simulink model "vdc_r2022a"  (R2022a)
settings: Solver=VariableStepAuto  StartTime=0.0  StopTime=10.0  RelTol=1e-3
libraries: simulink x1
settings Model: Creator=no  LastModifiedBy=no
settings ModelReferenceCC: EnableRefExpFcnMdlSchedulingChecks=off
settings RTWCC: Description=Generic Real-Time Target

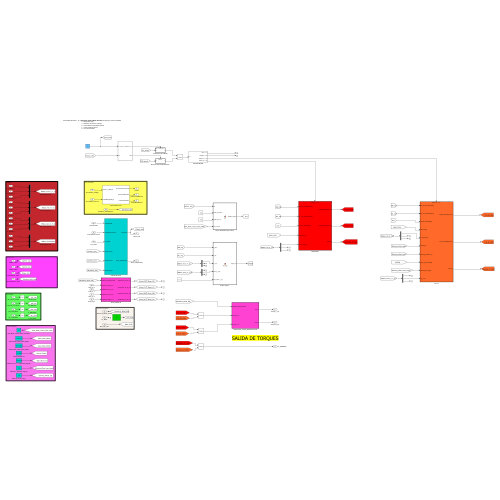
[thumbnail: Simulink's stored preview of the top-level diagram]
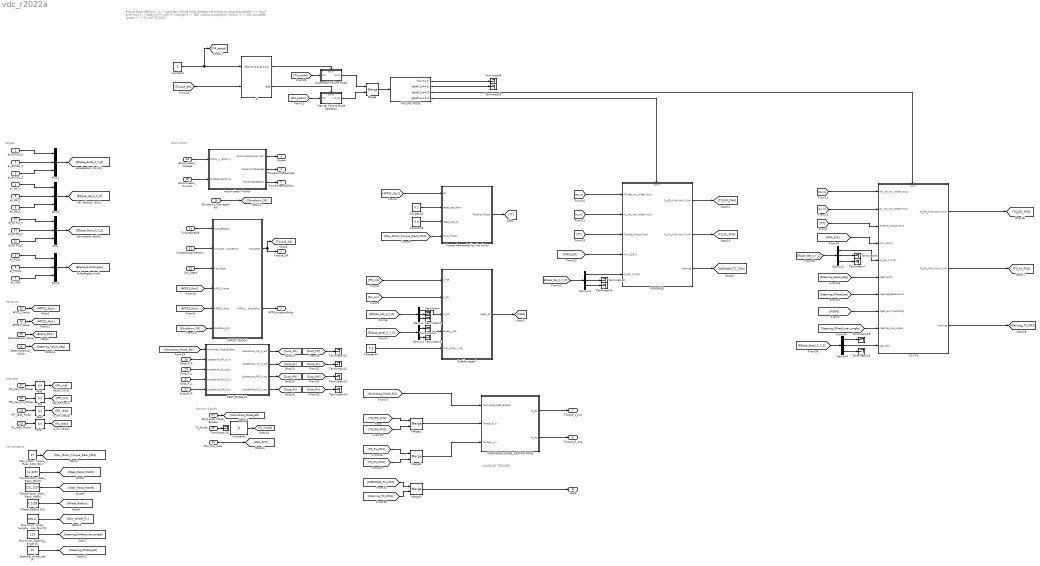
== system vdc_r2022a ==
  note: SALIDA DE TORQUES
  note: Ellipse
  note: Sensorics
  note: Velocities
  note: Car constants
  note: Failure Mode Selection: 5 -> Automatic Failure Mode Selection according to sensors available
      | 4 -> Rigid Axle (red)
      | 3 -> Steering TV with TC (orange)
      | 2 -> VDC without longitudinal (yellow)
      | 1 -> VDC complete (green)
      | 0 -> TV with TC 2023
  note: Accumulator
  note: Random Signals
  el_ACCEL_X : Inport
  el_ACCEL_Y : Inport  Port=2
  el_ACCEL_Z : Inport  Port=3
  el_Vel_X : Inport  Port=4
  el_Vel_Y : Inport  Port=5
  el_Vel_Z : Inport  Port=6
  el_YAW : Inport  Port=7
  el_PITCH : Inport  Port=8
  el_ROLL : Inport  Port=9
  el_GYRO_X : Inport  Port=10
  el_GYRO_Y : Inport  Port=11
  el_GYRO_Z : Inport  Port=12
  APPS2_Value : Inport  Port=13
  APPS1_Value : Inport  Port=14
  BrakeSensor_Value : Inport  Port=15
  SteeringSensor_Value : Inport  Port=16
  RL_Vel_ms_Wheel : Inport  Port=17
  RR_Vel_ms_Wheel : Inport  Port=18
  RR_rads_Motor : Inport  Port=19
  RL_rads_Motor : Inport  Port=20
  TorqueEnable : Inport  Port=21
  CriticalDisconnection : Inport  Port=22
  Car_State : Inport  Port=23
  Accumulator_Voltage : Inport  Port=24
  Accumulator_Current : Inport  Port=25
  Shutdown_PackageIntck : Inport  Port=26
  Workshop_Mode_Enable : Inport  Port=27
  TV_Mode : Inport  Port=28
  Susp_F_L : Inport  Port=29
  Susp_F_R : Inport  Port=30
  Susp_R_L : Inport  Port=31
  Susp_R_R : Inport  Port=32
  Max_slip_ratio : Inport  Port=33
  Abs{,1..3} (4 alike) : Abs  SaturateOnIntegerOverflow=off
  Accumulator Power : Subsystem
  Automatic Failure Mode : Subsystem  TreatAsAtomicUnit=on
  Constant : Constant  Value=5
  Constant1 : Constant  Value=3
  Constant2 : Constant  Value=0.2
  Constant3 : Constant  Value=0.8
  Constant4 : Constant  Value=7.5
  Demux{,1..4} (5 alike) : Demux  Outputs=3
  Enable regen? : MATLAB Function  TreatAsAtomicUnit=on
  FAILURE MODE : If  IfExpression=u1 == 1  ElseIfExpressions=u1 == 2, u1 == 3, u1 == 4  ShowElse=off
  If : If  NumInputs=2  IfExpression=u1 == 5 & u2 == 1
  Manual Failure Mode Selection : Subsystem  TreatAsAtomicUnit=on
  Max_Motor_Torque_Rear_FM4 [Nm] : Constant  Value=27
  Maximum_Force_Longitudinal_Slip [N] : Constant  Value=1364.44
  Maximum_Steering_angle [º] : Constant  Value=125
  Merge{,1..3} (4 alike) : Merge
  Mux{,1..3} (4 alike) : Mux  Inputs=3
  RIGIDAXLE : Subsystem
  SAFETY BLOCK : Subsystem
  Steering_wheel_sat [º] : Constant  Value=10
  TC+TV : Subsystem
  TEST_MODE_IN : Subsystem  TreatAsAtomicUnit=on
  Terminator{,1..16} (17 alike) : Terminator
  Torque demanded by the driver : MATLAB Function  TreatAsAtomicUnit=on
  Transmission_Gear_Ratio_MtoW : Constant  Value=11.3257
  Transmission_Gear_Ratio_WtoM : Constant  Value=1/11.3257
  WORKSHOP_MODE_RESTRICTIONS : Subsystem  TreatAsAtomicUnit=on
  Wheel_Radius [m] : Constant  Value=0.2285
  APPS_Implausibility : Outport  VectorParamsAs1DForOutWhenUnconnected=off
  Torque_OK : Outport  Port=2  VectorParamsAs1DForOutWhenUnconnected=off
  Power : Outport  Port=3  VectorParamsAs1DForOutWhenUnconnected=off
  PowerLimitReached : Outport  Port=4  VectorParamsAs1DForOutWhenUnconnected=off
  PowerMean500ms : Outport  Port=5  VectorParamsAs1DForOutWhenUnconnected=off
  Torque_R_out : Outport  Port=6
  Torque_L_out : Outport  Port=7
  Out3 : Outport  Port=8  SignalName=TC_WARNING
  wires:
  Torque demanded by the driver/1(Throttle_Torque) -> [TT]
  [TT] -> TC+TV/3(Throttle_Torque [Nm])
  Enable regen?/1(regen_en) -> [RGEN]
  [RGEN] -> TC+TV/8(regen_en [True/False])
  el_PITCH/1 -> Mux3/2
  el_GYRO_Z/1 -> Mux/3
  el_ACCEL_Y/1 -> Mux1/2
  Mux3/1 -> [Ellipse_EulerAngles]
  el_ROLL/1 -> Mux3/1
  Mux1/1 -> [Ellipse_Accel_X_Y_Z]
  el_YAW/1 -> Mux3/3
  el_Vel_X/1 -> Mux2/1
  Mux2/1 -> [Ellipse_Vel_X_Y_Z]
  el_GYRO_X/1 -> Mux/1
  el_Vel_Z/1 -> Mux2/3
  el_ACCEL_X/1 -> Mux1/1
  Mux/1 -> [Ellipse_Gyro_X_Y_Z]
  el_GYRO_Y/1 -> Mux/2
  el_ACCEL_Z/1 -> Mux1/3
  el_Vel_Y/1 -> Mux2/2
  SteeringSensor_Value/1 -> [Steering_Value_deg]
  APPS1_Value/1 -> [APPS1_0to1]
  BrakeSensor_Value/1 -> [Brake_0to1]
  APPS2_Value/1 -> [APPS2_0to1]
  [APPS1_0to1] -> Torque demanded by the driver/1(AP)
  Abs/1 -> [RR_ms]
  Abs2/1 -> [RR_rads]
  RR_Vel_ms_Wheel/1 -> Abs/1
  Abs1/1 -> [RL_ms]
  RR_rads_Motor/1 -> Abs2/1
  RL_rads_Motor/1 -> Abs3/1
  Abs3/1 -> [RL_rads]
  RL_Vel_ms_Wheel/1 -> Abs1/1
  Transmission_Gear_Ratio_MtoW/1 -> [Gear_Ratio_MtoW]
  Maximum_Force_Longitudinal_Slip [N]/1 -> [Max_Wheel_Fx]
  Transmission_Gear_Ratio_WtoM/1 -> [Gear_Ratio_WtoM]
  Wheel_Radius [m]/1 -> [Wheel_Radius]
  Max_Motor_Torque_Rear_FM4 [Nm]/1 -> [Max_Motor_Torque_Rear_FM4]
  [RR_ms] -> Enable regen?/1(V_RR)
  [RL_ms] -> Enable regen?/2(V_RL)
  [Ellipse_Vel_X_Y_Z] -> Demux/1
  Demux/1 -> Enable regen?/3(V_CG)
  Demux/2 -> Terminator/1
  Demux/3 -> Terminator1/1
  Demux1/3 -> Terminator3/1
  [Ellipse_Accel_X_Y_Z] -> Demux1/1
  Demux1/1 -> Terminator2/1
  Demux1/2 -> Enable regen?/4(accel_y_CG)
  [Max_Motor_Torque_Rear_FM4] -> Torque demanded by the driver/4(max_torque)
  Manual Failure Mode Selection/1(Out1) -> Merge/2
  If/2 -> Manual Failure Mode Selection/Action
  [FM_select] -> Manual Failure Mode Selection/1(In1)
  [TV_mode] -> Automatic Failure Mode/1(In1)
  Automatic Failure Mode/1(Out1) -> Merge/1
  Merge/1 -> FAILURE MODE/1
  Constant/1 -> [FM_select], If/1
  [APPS1_0to1] -> SAFETY BLOCK/4(APPS1_Value)
  SAFETY BLOCK/1(TorqueOK) -> Torque_OK/1, [Torque_OK]
  TorqueEnable/1 -> SAFETY BLOCK/1(TorqueEnable)
  SAFETY BLOCK/2(APPS_Implausibility) -> APPS_Implausibility/1
  [Shutdown_OK] -> SAFETY BLOCK/6(Shutdown_OK)
  [APPS2_0to1] -> SAFETY BLOCK/5(APPS2_Value)
  CriticalDisconnection/1 -> SAFETY BLOCK/2(CriticalDisconnection)
  Car_State/1 -> SAFETY BLOCK/3(Car_State)
  Accumulator Power/2(PowerLimitReached) -> PowerLimitReached/1
  Accumulator Power/1(AccumulatorPower [kW]) -> Power/1
  Accumulator Power/3(PowerMean500ms) -> PowerMean500ms/1
  Shutdown_PackageIntck/1 -> [Shutdown_OK]
  Accumulator_Voltage/1 -> Accumulator Power/1(TOTAL_V_BMS [V])
  Accumulator_Current/1 -> Accumulator Power/2(CURRENT_BMS [A])
  If/1 -> Automatic Failure Mode/Action
  FAILURE MODE/4 -> RIGIDAXLE/Action
  FAILURE MODE/3 -> TC+TV/Action
  FAILURE MODE/2 -> Terminator5/1
  FAILURE MODE/1 -> Terminator4/1
  Maximum_Steering_angle [º]/1 -> [Steering_Wheel_max_angle]
  Steering_wheel_sat [º]/1 -> [Steering_Wheel_sat]
  [Torque_OK] -> If/2
  [RR_ms] -> TC+TV/1(RR_Vel_ms_Wheel [m/s])
  [RL_ms] -> TC+TV/2(RL_Vel_ms_Wheel [m/s])
  [MAX_SLR] -> TC+TV/4(MAX_SLR [])
  [Steering_Value_deg] -> TC+TV/6(steering (º))
  [Steering_Wheel_sat] -> TC+TV/7(steering_deadzone (º))
  [Ellipse_Vel_X_Y_Z] -> Demux2/1
  Demux2/1 -> TC+TV/5(el_Vel_X [m/s])
  Demux2/2 -> Terminator6/1
  Demux2/3 -> Terminator7/1
  Demux3/3 -> Terminator9/1
  Demux3/2 -> Terminator8/1
  [Ellipse_Vel_X_Y_Z] -> Demux3/1
  Demux3/1 -> RIGIDAXLE/5(el_Vel_X [m/s])
  [RR_ms] -> RIGIDAXLE/1(RR_Vel_ms_Wheel [m/s])
  [TT] -> RIGIDAXLE/3(Throttle_Torque [Nm])
  [RL_ms] -> RIGIDAXLE/2(RL_Vel_ms_Wheel [m/s])
  [MAX_SLR] -> RIGIDAXLE/4(MAX_SLR [])
  RIGIDAXLE/1(Tq_RR_FM4 [Nm] (0,inf)) -> [TQ_RR_FM4]
  RIGIDAXLE/2(Tq_RL_FM4 [Nm] (0,inf)) -> [TQ_RL_FM4]
  TC+TV/1(Tq_RR_FM3 [Nm] (0,inf)) -> [TQ_RR_FM3]
  TC+TV/2(Tq_RL_FM3 [Nm] (0,inf)) -> [TQ_RL_FM3]
  [TQ_RR_FM4] -> Merge1/1
  [TQ_RR_FM3] -> Merge1/2
  [TQ_RL_FM4] -> Merge2/1
  [TQ_RL_FM3] -> Merge2/2
  Constant1/1 -> [TV_mode]
  Workshop_Mode_Enable/1 -> [Workshop_Mode_EN]
  TV_Mode/1 -> Terminator10/1
  TEST_MODE_IN/2(Suspension_FL_N_out) -> [Susp_FL]
  [Workshop_Mode_EN] -> TEST_MODE_IN/1(Workshop_Mode_Enable)
  Susp_F_R/1 -> TEST_MODE_IN/2(Suspension_FR_N_in)
  Susp_R_L/1 -> TEST_MODE_IN/4(Suspension_RL_N_in)
  Susp_R_R/1 -> TEST_MODE_IN/5(Suspension_RR_N_in)
  TEST_MODE_IN/3(Suspension_RR_N_out) -> [Susp_RR]
  Susp_F_L/1 -> TEST_MODE_IN/3(Suspension_FL_N_in)
  TEST_MODE_IN/4(Suspension_RL_N_out) -> [Susp_RL]
  TEST_MODE_IN/1(Suspension_FR_N_out) -> [Susp_FR]
  [Susp_FR] -> Terminator11/1
  [Susp_RL] -> Terminator14/1
  [Susp_RR] -> Terminator13/1
  [Susp_FL] -> Terminator12/1
  Constant2/1 -> Torque demanded by the driver/2(pedal_sat_down)
  Constant3/1 -> Torque demanded by the driver/3(pedal_sat_up)
  Constant4/1 -> Enable regen?/5(max_accel_y_cg)
  [Steering_Wheel_max_angle] -> TC+TV/9(steering_max_angle)
  RIGIDAXLE/3(warning) -> [WARNING_TC_FM4]
  [WARNING_TC_FM4] -> Merge3/1
  Merge3/1 -> Out3/1
  TC+TV/3(warning) -> [Warning_TC_FM3]
  [Warning_TC_FM3] -> Merge3/2
  WORKSHOP_MODE_RESTRICTIONS/1(Tq_RL) -> Torque_L_out/1
  WORKSHOP_MODE_RESTRICTIONS/2(Tq_RR) -> Torque_R_out/1
  Merge1/1 -> WORKSHOP_MODE_RESTRICTIONS/2(Torque_R_in)
  Merge2/1 -> WORKSHOP_MODE_RESTRICTIONS/3(Torque_L_in)
  [Workshop_Mode_EN] -> WORKSHOP_MODE_RESTRICTIONS/1(Workshop_Mode_Enable)
  Demux4/3 -> Terminator16/1
  Demux4/1 -> Terminator15/1
  [Ellipse_Accel_X_Y_Z] -> Demux4/1
  Demux4/2 -> TC+TV/10(cg_y_acc)
  Max_slip_ratio/1 -> [MAX_SLR]

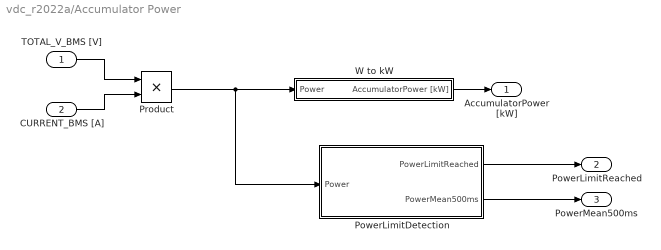
== system vdc_r2022a/Accumulator Power ==
  TOTAL_V_BMS [V] : Inport
  CURRENT_BMS [A] : Inport  Port=2
  PowerLimitDetection : Subsystem  TreatAsAtomicUnit=on
  Product : Product
  W to kW : Subsystem
  AccumulatorPower [kW] : Outport  VectorParamsAs1DForOutWhenUnconnected=off
  PowerLimitReached : Outport  Port=2  VectorParamsAs1DForOutWhenUnconnected=off
  PowerMean500ms : Outport  Port=3  VectorParamsAs1DForOutWhenUnconnected=off
  wires:
  Product/1 -> W to kW/1(Power), PowerLimitDetection/1(Power)
  PowerLimitDetection/1(PowerLimitReached) -> PowerLimitReached/1
  PowerLimitDetection/2(PowerMean500ms) -> PowerMean500ms/1
  TOTAL_V_BMS [V]/1 -> Product/1
  CURRENT_BMS [A]/1 -> Product/2
  W to kW/1(AccumulatorPower [kW]) -> AccumulatorPower [kW]/1

== system vdc_r2022a/Automatic Failure Mode ==
  In1 : Inport
  Action Port : ActionPort  ActionPortLabel=if(u1 == 5 & u2 == 1)
  Out1 : Outport  VectorParamsAs1DForOutWhenUnconnected=off
  wires:
  In1/1 -> Out1/1

== system vdc_r2022a/Manual Failure Mode Selection ==
  In1 : Inport
  Action Port : ActionPort  ActionPortLabel=else
  Out1 : Outport  VectorParamsAs1DForOutWhenUnconnected=off
  wires:
  In1/1 -> Out1/1

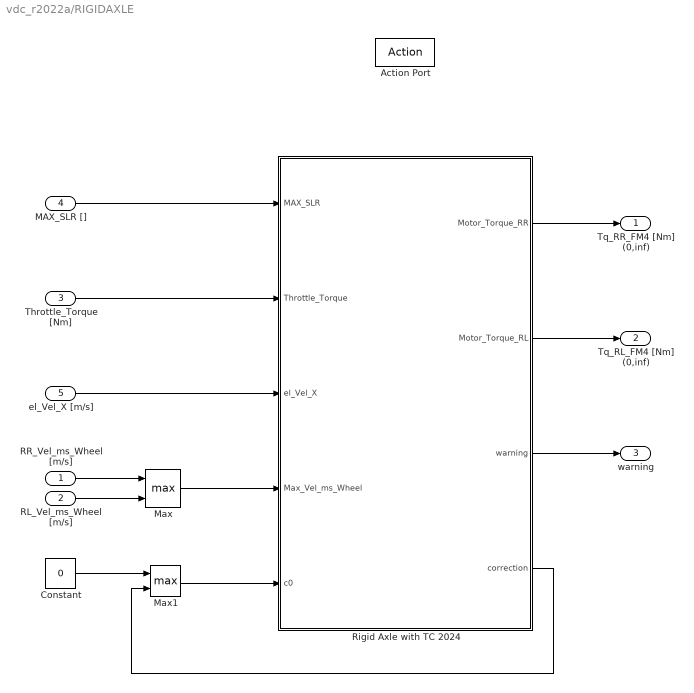
== system vdc_r2022a/RIGIDAXLE ==
  RR_Vel_ms_Wheel [m/s] : Inport
  RL_Vel_ms_Wheel [m/s] : Inport  Port=2
  Throttle_Torque [Nm] : Inport  Port=3
  MAX_SLR [] : Inport  Port=4
  el_Vel_X [m/s] : Inport  Port=5
  Action Port : ActionPort  ActionPortLabel=elseif( u1 == 4)
  Constant : Constant  Value=0
  Max : MinMax  Function=max  Inputs=2
  Max1 : MinMax  Function=max  Inputs=2
  "Rigid Axle with TC 2024 " : MATLAB Function  TreatAsAtomicUnit=on
  Tq_RR_FM4 [Nm] (0,inf) : Outport  VectorParamsAs1DForOutWhenUnconnected=off
  Tq_RL_FM4 [Nm] (0,inf) : Outport  Port=2  VectorParamsAs1DForOutWhenUnconnected=off
  warning : Outport  Port=3
  wires:
  RR_Vel_ms_Wheel [m/s]/1 -> Max/1
  "Rigid Axle with TC 2024 "/1(Motor_Torque_RR) -> Tq_RR_FM4 [Nm] (0,inf)/1
  "Rigid Axle with TC 2024 "/4(correction) -> Max1/2
  Constant/1 -> Max1/1
  Max1/1 -> "Rigid Axle with TC 2024 "/5(c0)
  "Rigid Axle with TC 2024 "/2(Motor_Torque_RL) -> Tq_RL_FM4 [Nm] (0,inf)/1
  Max/1 -> "Rigid Axle with TC 2024 "/4(Max_Vel_ms_Wheel)
  RL_Vel_ms_Wheel [m/s]/1 -> Max/2
  Throttle_Torque [Nm]/1 -> "Rigid Axle with TC 2024 "/2(Throttle_Torque)
  MAX_SLR []/1 -> "Rigid Axle with TC 2024 "/1(MAX_SLR)
  el_Vel_X [m/s]/1 -> "Rigid Axle with TC 2024 "/3(el_Vel_X)
  "Rigid Axle with TC 2024 "/3(warning) -> warning/1

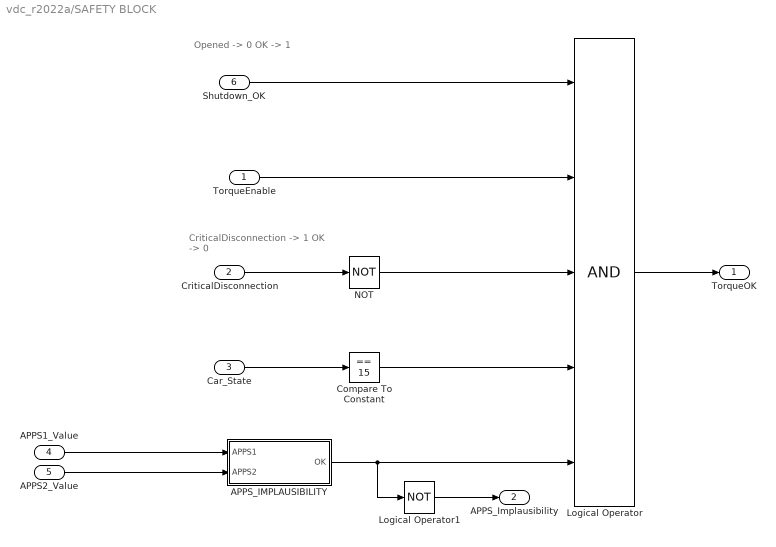
== system vdc_r2022a/SAFETY BLOCK ==
  note: CriticalDisconnection -> 1
      | OK -> 0
  note: Opened -> 0
      | OK -> 1
  TorqueEnable : Inport
  CriticalDisconnection : Inport  Port=2
  Car_State : Inport  Port=3
  APPS1_Value : Inport  Port=4
  APPS2_Value : Inport  Port=5
  Shutdown_OK : Inport  Port=6
  APPS_IMPLAUSIBILITY : Subsystem
  Compare To Constant : simulink/Logic and Bit Operations/Compare To Constant  relop===  const=15  OutDataTypeStr=boolean
  Logical Operator : Logic  Inputs=5  OutDataTypeStr=boolean
  Logical Operator1 : Logic  Operator=NOT  IconShape=distinctive  AllPortsSameDT=off  OutDataTypeStr=boolean
  NOT : Logic  Operator=NOT  IconShape=distinctive  AllPortsSameDT=off  OutDataTypeStr=boolean
  TorqueOK : Outport  VectorParamsAs1DForOutWhenUnconnected=off
  APPS_Implausibility : Outport  Port=2  VectorParamsAs1DForOutWhenUnconnected=off
  wires:
  Logical Operator/1 -> TorqueOK/1
  Car_State/1 -> Compare To Constant/1
  NOT/1 -> Logical Operator/3
  CriticalDisconnection/1 -> NOT/1
  TorqueEnable/1 -> Logical Operator/2
  APPS2_Value/1 -> APPS_IMPLAUSIBILITY/2(APPS2)
  APPS1_Value/1 -> APPS_IMPLAUSIBILITY/1(APPS1)
  Logical Operator1/1 -> APPS_Implausibility/1
  Compare To Constant/1 -> Logical Operator/4
  APPS_IMPLAUSIBILITY/1(OK) -> Logical Operator/5, Logical Operator1/1
  Shutdown_OK/1 -> Logical Operator/1

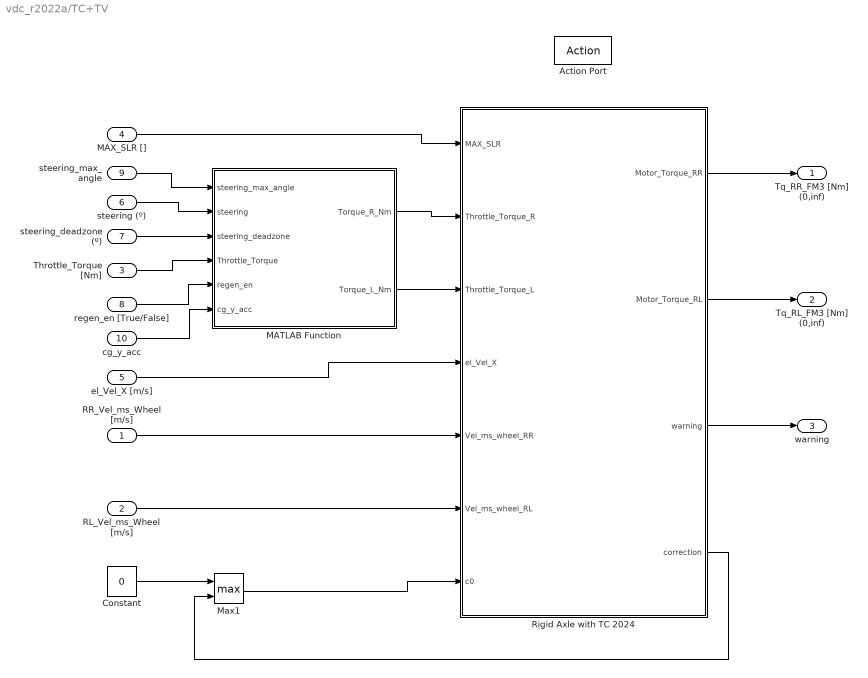
== system vdc_r2022a/TC+TV ==
  RR_Vel_ms_Wheel [m/s] : Inport
  RL_Vel_ms_Wheel [m/s] : Inport  Port=2
  Throttle_Torque [Nm] : Inport  Port=3
  MAX_SLR [] : Inport  Port=4
  el_Vel_X [m/s] : Inport  Port=5
  steering (º) : Inport  Port=6
  steering_deadzone (º) : Inport  Port=7
  regen_en [True/False] : Inport  Port=8
  steering_max_angle : Inport  Port=9
  cg_y_acc : Inport  Port=10
  Action Port : ActionPort  ActionPortLabel=elseif( u1 == 3)
  Constant : Constant  Value=0
  MATLAB Function : MATLAB Function  TreatAsAtomicUnit=on
  Max1 : MinMax  Function=max  Inputs=2
  "Rigid Axle with TC 2024 " : MATLAB Function  TreatAsAtomicUnit=on
  Tq_RR_FM3 [Nm] (0,inf) : Outport  VectorParamsAs1DForOutWhenUnconnected=off
  Tq_RL_FM3 [Nm] (0,inf) : Outport  Port=2  VectorParamsAs1DForOutWhenUnconnected=off
  warning : Outport  Port=3
  wires:
  RR_Vel_ms_Wheel [m/s]/1 -> "Rigid Axle with TC 2024 "/5(Vel_ms_wheel_RR)
  "Rigid Axle with TC 2024 "/1(Motor_Torque_RR) -> Tq_RR_FM3 [Nm] (0,inf)/1
  "Rigid Axle with TC 2024 "/4(correction) -> Max1/2
  Constant/1 -> Max1/1
  Max1/1 -> "Rigid Axle with TC 2024 "/7(c0)
  "Rigid Axle with TC 2024 "/2(Motor_Torque_RL) -> Tq_RL_FM3 [Nm] (0,inf)/1
  RL_Vel_ms_Wheel [m/s]/1 -> "Rigid Axle with TC 2024 "/6(Vel_ms_wheel_RL)
  Throttle_Torque [Nm]/1 -> MATLAB Function/4(Throttle_Torque)
  MATLAB Function/1(Torque_R_Nm) -> "Rigid Axle with TC 2024 "/2(Throttle_Torque_R)
  MATLAB Function/2(Torque_L_Nm) -> "Rigid Axle with TC 2024 "/3(Throttle_Torque_L)
  MAX_SLR []/1 -> "Rigid Axle with TC 2024 "/1(MAX_SLR)
  el_Vel_X [m/s]/1 -> "Rigid Axle with TC 2024 "/4(el_Vel_X)
  steering (º)/1 -> MATLAB Function/2(steering)
  steering_deadzone (º)/1 -> MATLAB Function/3(steering_deadzone)
  regen_en [True/False]/1 -> MATLAB Function/5(regen_en)
  steering_max_angle/1 -> MATLAB Function/1(steering_max_angle)
  "Rigid Axle with TC 2024 "/3(warning) -> warning/1
  cg_y_acc/1 -> MATLAB Function/6(cg_y_acc)

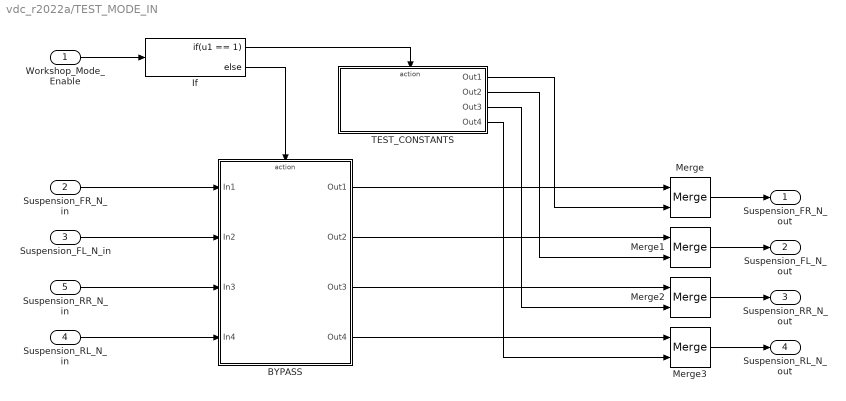
== system vdc_r2022a/TEST_MODE_IN ==
  Workshop_Mode_Enable : Inport
  Suspension_FR_N_in : Inport  Port=2
  Suspension_FL_N_in : Inport  Port=3
  Suspension_RL_N_in : Inport  Port=4
  Suspension_RR_N_in : Inport  Port=5
  BYPASS : Subsystem  TreatAsAtomicUnit=on
  If : If  IfExpression=u1 == 1
  Merge{,1..3} (4 alike) : Merge
  TEST_CONSTANTS : Subsystem  TreatAsAtomicUnit=on
  Suspension_FR_N_out : Outport  VectorParamsAs1DForOutWhenUnconnected=off
  Suspension_FL_N_out : Outport  Port=2  VectorParamsAs1DForOutWhenUnconnected=off
  Suspension_RR_N_out : Outport  Port=3  VectorParamsAs1DForOutWhenUnconnected=off
  Suspension_RL_N_out : Outport  Port=4  VectorParamsAs1DForOutWhenUnconnected=off
  wires:
  Suspension_FR_N_in/1 -> BYPASS/1(In1)
  Suspension_FL_N_in/1 -> BYPASS/2(In2)
  Suspension_RR_N_in/1 -> BYPASS/3(In3)
  Suspension_RL_N_in/1 -> BYPASS/4(In4)
  Merge/1 -> Suspension_FR_N_out/1
  Merge1/1 -> Suspension_FL_N_out/1
  Merge2/1 -> Suspension_RR_N_out/1
  Merge3/1 -> Suspension_RL_N_out/1
  BYPASS/1(Out1) -> Merge/1
  BYPASS/2(Out2) -> Merge1/1
  BYPASS/3(Out3) -> Merge2/1
  BYPASS/4(Out4) -> Merge3/1
  Workshop_Mode_Enable/1 -> If/1
  If/2 -> BYPASS/Action
  If/1 -> TEST_CONSTANTS/Action
  TEST_CONSTANTS/4(Out4) -> Merge3/2
  TEST_CONSTANTS/3(Out3) -> Merge2/2
  TEST_CONSTANTS/2(Out2) -> Merge1/2
  TEST_CONSTANTS/1(Out1) -> Merge/2

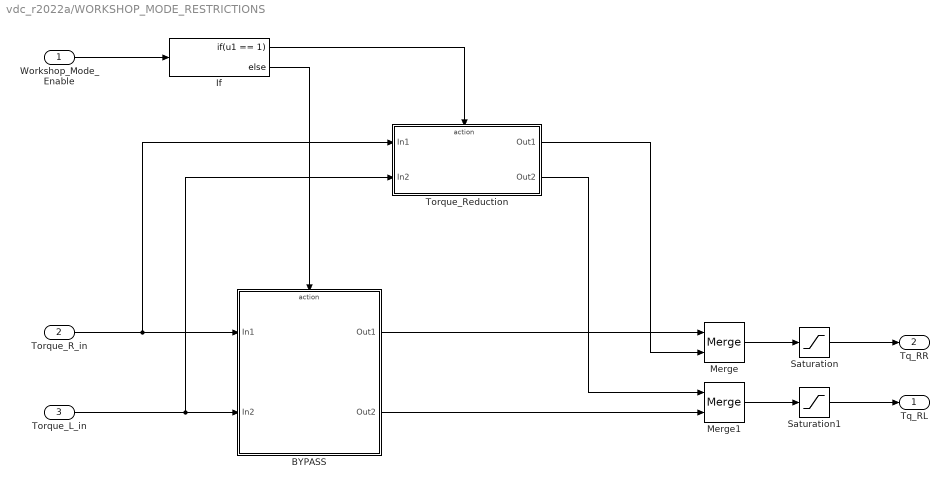
== system vdc_r2022a/WORKSHOP_MODE_RESTRICTIONS ==
  Workshop_Mode_Enable : Inport
  Torque_R_in : Inport  Port=2
  Torque_L_in : Inport  Port=3
  BYPASS : Subsystem  TreatAsAtomicUnit=on
  If : If  IfExpression=u1 == 1
  Merge : Merge
  Merge1 : Merge
  Saturation : Saturate  UpperLimit=580  LowerLimit=-580
  Saturation1 : Saturate  UpperLimit=580  LowerLimit=-580
  "Torque_Reduction " : Subsystem  TreatAsAtomicUnit=on
  Tq_RL : Outport  VectorParamsAs1DForOutWhenUnconnected=off
  Tq_RR : Outport  Port=2  VectorParamsAs1DForOutWhenUnconnected=off
  wires:
  If/2 -> BYPASS/Action
  If/1 -> "Torque_Reduction "/Action
  Workshop_Mode_Enable/1 -> If/1
  Torque_R_in/1 -> "Torque_Reduction "/1(In1), BYPASS/1(In1)
  Torque_L_in/1 -> "Torque_Reduction "/2(In2), BYPASS/2(In2)
  BYPASS/1(Out1) -> Merge/1
  BYPASS/2(Out2) -> Merge1/2
  "Torque_Reduction "/1(Out1) -> Merge/2
  "Torque_Reduction "/2(Out2) -> Merge1/1
  Merge/1 -> Saturation/1
  Merge1/1 -> Saturation1/1
  Saturation/1 -> Tq_RR/1
  Saturation1/1 -> Tq_RL/1

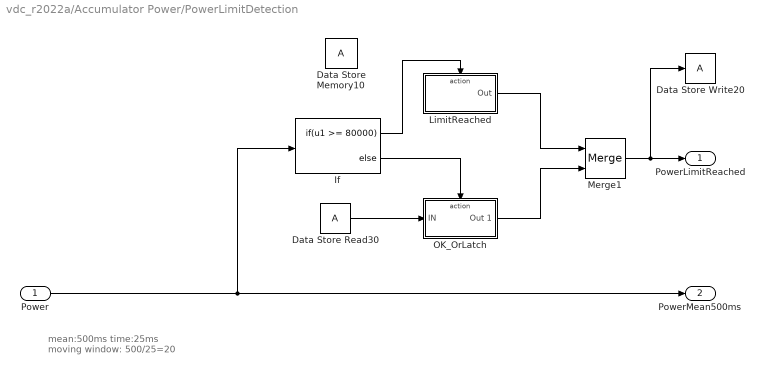
== system vdc_r2022a/Accumulator Power/PowerLimitDetection ==
  note: mean:500ms
      | time:25ms
      | moving window: 500/25=20
  Power : Inport
  Data Store Memory10 : DataStoreMemory  ReadBeforeWriteMsg=warning  WriteAfterWriteMsg=warning  WriteAfterReadMsg=warning  ShowAdditionalParam=off
  Data Store Read30 : DataStoreRead  IndexOptions=Index vector (dialog)  Indices=1  OutputSizes=1
  Data Store Write20 : DataStoreWrite  IndexOptions=Index vector (dialog)  Indices=1  OutputSizes=1
  If : If  IfExpression=u1 >= 80000
  LimitReached : Subsystem  TreatAsAtomicUnit=on
  Merge1 : Merge
  OK_OrLatch : Subsystem  TreatAsAtomicUnit=on
  PowerLimitReached : Outport  VectorParamsAs1DForOutWhenUnconnected=off
  PowerMean500ms : Outport  Port=2  VectorParamsAs1DForOutWhenUnconnected=off
  wires:
  Power/1 -> If/1, PowerMean500ms/1
  If/1 -> LimitReached/Action
  If/2 -> OK_OrLatch/Action
  LimitReached/1("Out ") -> Merge1/1
  OK_OrLatch/1(Out 1) -> Merge1/2
  Merge1/1 -> Data Store Write20/1, PowerLimitReached/1
  Data Store Read30/1 -> OK_OrLatch/1(IN)

== system vdc_r2022a/Accumulator Power/W to kW ==
  Power : Inport
  0-100 to 0-2 : Constant  Value=1000
  Divide5 : Product  Inputs=*/
  AccumulatorPower [kW] : Outport  VectorParamsAs1DForOutWhenUnconnected=off
  wires:
  Power/1 -> Divide5/1
  0-100 to 0-2/1 -> Divide5/2
  Divide5/1 -> AccumulatorPower [kW]/1

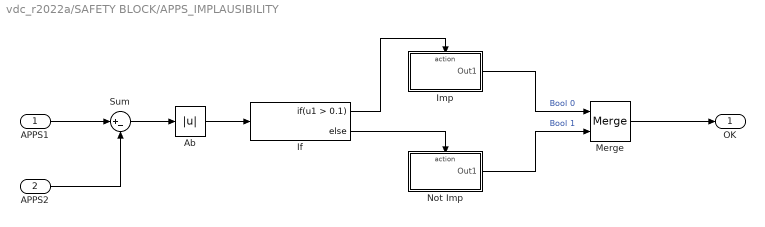
== system vdc_r2022a/SAFETY BLOCK/APPS_IMPLAUSIBILITY ==
  APPS1 : Inport
  APPS2 : Inport  Port=2
  Ab : Abs  SaturateOnIntegerOverflow=off
  If : If  IfExpression=u1 > 0.1
  Imp : Subsystem  TreatAsAtomicUnit=on
  Merge : Merge
  Not Imp : Subsystem  TreatAsAtomicUnit=on
  Sum : Sum  Inputs=|+-
  OK : Outport  VectorParamsAs1DForOutWhenUnconnected=off
  wires:
  APPS1/1 -> Sum/1
  APPS2/1 -> Sum/2
  Sum/1 -> Ab/1
  Ab/1 -> If/1
  Imp/1(Out1) -> Merge/1  "Bool 0"
  Not Imp/1(Out1) -> Merge/2  "Bool 1"
  Merge/1 -> OK/1
  If/2 -> Not Imp/Action
  If/1 -> Imp/Action

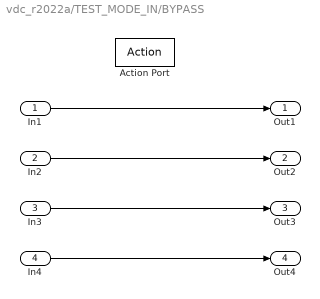
== system vdc_r2022a/TEST_MODE_IN/BYPASS ==
  In1 : Inport
  In2 : Inport  Port=2
  In3 : Inport  Port=3
  In4 : Inport  Port=4
  Action Port : ActionPort
  Out1 : Outport  VectorParamsAs1DForOutWhenUnconnected=off
  Out2 : Outport  Port=2  VectorParamsAs1DForOutWhenUnconnected=off
  Out3 : Outport  Port=3  VectorParamsAs1DForOutWhenUnconnected=off
  Out4 : Outport  Port=4  VectorParamsAs1DForOutWhenUnconnected=off
  wires:
  In1/1 -> Out1/1
  In2/1 -> Out2/1
  In3/1 -> Out3/1
  In4/1 -> Out4/1

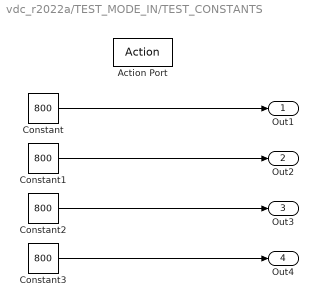
== system vdc_r2022a/TEST_MODE_IN/TEST_CONSTANTS ==
  Action Port : ActionPort
  Constant{,1..3} (4 alike) : Constant  Value=800
  Out1 : Outport  VectorParamsAs1DForOutWhenUnconnected=off
  Out2 : Outport  Port=2  VectorParamsAs1DForOutWhenUnconnected=off
  Out3 : Outport  Port=3  VectorParamsAs1DForOutWhenUnconnected=off
  Out4 : Outport  Port=4  VectorParamsAs1DForOutWhenUnconnected=off
  wires:
  Constant/1 -> Out1/1
  Constant1/1 -> Out2/1
  Constant2/1 -> Out3/1
  Constant3/1 -> Out4/1

== system vdc_r2022a/WORKSHOP_MODE_RESTRICTIONS/BYPASS ==
  In1 : Inport
  In2 : Inport  Port=2
  Action Port : ActionPort
  Out1 : Outport  VectorParamsAs1DForOutWhenUnconnected=off
  Out2 : Outport  Port=2  VectorParamsAs1DForOutWhenUnconnected=off
  wires:
  In1/1 -> Out1/1
  In2/1 -> Out2/1

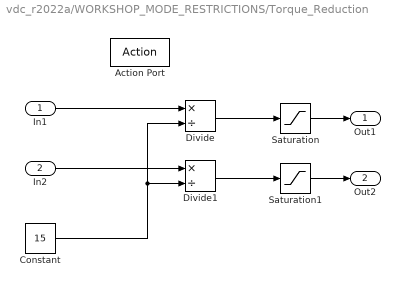
== system vdc_r2022a/WORKSHOP_MODE_RESTRICTIONS/Torque_Reduction  ==
  In1 : Inport
  In2 : Inport  Port=2
  Action Port : ActionPort
  Constant : Constant  Value=15
  Divide : Product  Inputs=*/
  Divide1 : Product  Inputs=*/
  Saturation : Saturate  UpperLimit=10  LowerLimit=-10
  Saturation1 : Saturate  UpperLimit=10  LowerLimit=-10
  Out1 : Outport  VectorParamsAs1DForOutWhenUnconnected=off
  Out2 : Outport  Port=2  VectorParamsAs1DForOutWhenUnconnected=off
  wires:
  Saturation/1 -> Out1/1
  Saturation1/1 -> Out2/1
  In1/1 -> Divide/1
  Divide/1 -> Saturation/1
  In2/1 -> Divide1/1
  Divide1/1 -> Saturation1/1
  Constant/1 -> Divide1/2, Divide/2

== system vdc_r2022a/Accumulator Power/PowerLimitDetection/LimitReached ==
  Action Port : ActionPort
  Constant : Constant
  "Out " : Outport  VectorParamsAs1DForOutWhenUnconnected=off
  wires:
  Constant/1 -> "Out "/1

== system vdc_r2022a/Accumulator Power/PowerLimitDetection/OK_OrLatch ==
  IN : Inport
  Action Port : ActionPort
  If : If  IfExpression=(u1>0)
  Latched Error : Subsystem  TreatAsAtomicUnit=on
  Merge : Merge
  OK : Subsystem  TreatAsAtomicUnit=on
  Out 1 : Outport  VectorParamsAs1DForOutWhenUnconnected=off
  wires:
  IN/1 -> If/1
  If/1 -> Latched Error/Action
  If/2 -> OK/Action
  Latched Error/1("Out ") -> Merge/1
  OK/1("Out ") -> Merge/2
  Merge/1 -> Out 1/1

== system vdc_r2022a/SAFETY BLOCK/APPS_IMPLAUSIBILITY/Imp ==
  Action Port : ActionPort
  Constant : Constant  Value=0  OutDataTypeStr=boolean
  Out1 : Outport  VectorParamsAs1DForOutWhenUnconnected=off
  wires:
  Constant/1 -> Out1/1  "Boolean"

== system vdc_r2022a/SAFETY BLOCK/APPS_IMPLAUSIBILITY/Not Imp ==
  Action Port : ActionPort
  Constant : Constant  OutDataTypeStr=boolean
  Out1 : Outport  VectorParamsAs1DForOutWhenUnconnected=off
  wires:
  Constant/1 -> Out1/1  "Boolean"

== system vdc_r2022a/Accumulator Power/PowerLimitDetection/OK_OrLatch/Latched Error ==
  Action Port : ActionPort
  Constant : Constant
  "Out " : Outport  VectorParamsAs1DForOutWhenUnconnected=off
  wires:
  Constant/1 -> "Out "/1

== system vdc_r2022a/Accumulator Power/PowerLimitDetection/OK_OrLatch/OK ==
  Action Port : ActionPort
  Constant : Constant  Value=0
  "Out " : Outport  VectorParamsAs1DForOutWhenUnconnected=off
  wires:
  Constant/1 -> "Out "/1

== matlab function vdc_r2022a/Torque demanded by the driver ==
  data: Throttle_Torque output; AP input; pedal_sat_down input; pedal_sat_up input; max_torque input
function Throttle_Torque  = TT(AP, pedal_sat_down, pedal_sat_up, max_torque)
if AP <= pedal_sat_down %establish the lower deadzone for the throttle pedal
    Throttle_Response = 0;
end
if AP >= pedal_sat_up %establish the higher deadzone for the throttle pedal
    Throttle_Response = 1;
end
if AP >= pedal_sat_down && AP <= pedal_sat_up
    Throttle_Response = (AP-pedal_sat_down/pedal_sat_up-pedal_sat_down); %evaluate for given input
end
Throttle_Torque = Throttle_Response * max_torque; % set torque to max output times pedal factor
end

== matlab function vdc_r2022a/TC+TV/Rigid Axle with TC 2024  ==
  data: MAX_SLR input; Throttle_Torque_R input; Throttle_Torque_L input; Motor_Torque_RR output; Motor_Torque_RL output; warning output; el_Vel_X input; Vel_ms_wheel_RR input; Vel_ms_wheel_RL input; correction output; c0 input
function [Motor_Torque_RR, Motor_Torque_RL, warning,correction] = RigidAxle_TC_2024(MAX_SLR, Throttle_Torque_R, Throttle_Torque_L, el_Vel_X, Vel_ms_wheel_RR, Vel_ms_wheel_RL, c0)

% SLIP RATIO CALCULATIONS
    % calculate slip ratio
    SLR_RR = (Vel_ms_wheel_RR/el_Vel_X);
    SLR_RL = (Vel_ms_wheel_RL/el_Vel_X);

% CHECK FOR EXCESIVE SLIPPING
    % SLIP RATIO LESSER THAN MAXIMUM SLIP RATIO => apply max torque times throttle factor
        if(SLR_RR<MAX_SLR)
            Motor_Torque_RR = Throttle_Torque_R; 
            correction = 0; %set correction to 0 as tyre is not slipping
            warning = false;
        else
            warning = true;
        % TYRE SLIPPING => TC INTERVENES
            % LOOK FOR THE PREVIOUS CORRECTION [Nm]
            if(c0 == 0) % NOT SLIPPING PREVIOUSLY
                correction = 1; % [INTERVAL TO BE DETERMINED] set the correction to the torque we want to substract
                Motor_Torque_RR = Throttle_Torque_R-correction; % substract the correction from the torque to apply
            else % TYRE SLIPPING PREVIOUSLY
                correction = c0 + 1; % [INTERVAL TO BE DETERMINED] set the correction to the torque we want to substract + previous corrections
                Motor_Torque_RR = Throttle_Torque_R-correction; % substract the correction from the torque to apply
            end
        end

% CHECK FOR EXCESIVE SLIPPING
    % SLIP RATIO LESSER THAN MAXIMUM SLIP RATIO => apply max torque times throttle factor
        if(SLR_RL<MAX_SLR)
            Motor_Torque_RL = Throttle_Torque_L;
            correction = 0; %set correction to 0 as tyre is not slipping
        else
            warning = true;
        % TYRE SLIPPING => TC INTERVENES
            % LOOK FOR THE PREVIOUS CORRECTION [Nm]
            if(c0 == 0) % NOT SLIPPING PREVIOUSLY
                correction = 1; % [INTERVAL TO BE DETERMINED] set the correction to the torque we want to substract
                Motor_Torque_RL = Throttle_Torque_L-correction; % substract the correction from the torque to apply
            else % TYRE SLIPPING PREVIOUSLY
                correction = c0 + 1; % [INTERVAL TO BE DETERMINED] set the correction to the torque we want to substract + previous corrections
                Motor_Torque_RL = Throttle_Torque_L-correction; % substract the correction from the torque to apply
            end
        end
end

== matlab function vdc_r2022a/RIGIDAXLE/Rigid Axle with TC 2024  ==
  data: MAX_SLR input; Throttle_Torque input; Motor_Torque_RR output; Motor_Torque_RL output; warning output; el_Vel_X input; Max_Vel_ms_Wheel input; correction output; c0 input
function [Motor_Torque_RR, Motor_Torque_RL, warning, correction] = RigidAxle_TC_2024(MAX_SLR, Throttle_Torque, el_Vel_X, Max_Vel_ms_Wheel, c0)

% SLIP RATIO CALCULATIONS
    % calculate slip ratio
    SLR = (Max_Vel_ms_Wheel/el_Vel_X);

% CHECK FOR EXCESIVE SLIPPING
    % SLIP RATIO LESSER THAN MAXIMUM SLIP RATIO => apply max torque times throttle factor
        if(SLR<MAX_SLR)
            Motor_Torque_RR = Throttle_Torque; 
            Motor_Torque_RL = Throttle_Torque;
            correction = 0; %set correction to 0 as tyre is not slipping
            warning = false;
            return;
        else
            warning = true;
        % TYRE SLIPPING => TC INTERVENES
            % LOOK FOR THE PREVIOUS CORRECTION [Nm]
            if(c0 == 0) % NOT SLIPPING PREVIOUSLY
                correction = 1; % [INTERVAL TO BE DETERMINED] set the correction to the torque we want to substract
                Motor_Torque_RR = Throttle_Torque-correction; % substract the correction from the torque to apply
                Motor_Torque_RL = Throttle_Torque-correction;
                return;
            else % TYRE SLIPPING PREVIOUSLY
                correction = c0 + 1; % [INTERVAL TO BE DETERMINED] set the correction to the torque we want to substract + previous corrections
                Motor_Torque_RR = Throttle_Torque-correction; % substract the correction from the torque to apply
                Motor_Torque_RL = Throttle_Torque-correction;
                return;
            end
        end
end

== matlab function vdc_r2022a/TC+TV/MATLAB Function ==
  data: steering_max_angle input; Torque_R_Nm output; Torque_L_Nm output; steering input; steering_deadzone input; Throttle_Torque input; regen_en input; cg_y_acc input
function [Torque_R_Nm, Torque_L_Nm] = TV(steering_max_angle, steering, steering_deadzone, Throttle_Torque, regen_en, cg_y_acc)

if abs(steering)<=steering_deadzone %add steering deadzone (º)
    Torque_L_Nm = Throttle_Torque;
    Torque_R_Nm = Throttle_Torque;
    return;
end
if(steering/cg_y_acc > 0) % check for driver correcting oversteer to avoid overcorrecting
    Torque_L_Nm = Throttle_Torque;
    Torque_R_Nm = Throttle_Torque;
    return;
end
d = (abs(steering)-steering_deadzone)/(steering_max_angle-steering_deadzone); %evaluate delta torque for given steering angle

if d>Throttle_Torque && regen_en ~= true
    d=torque;%force torque to be positive to avoid balance issues
end
if s<0 %if steering left, apply full torque to the emotor on the outside
       %and substract the delta from the inside one
    Torque_L_Nm = Throttle_Torque-d;
    Torque_R_Nm = Throttle_Torque;
    return;
end
%opposite case
Torque_L_Nm = Throttle_Torque;
Torque_R_Nm = Throttle_Torque-d;
end

== matlab function vdc_r2022a/Enable regen? ==
  data: V_RR input; regen_en output; V_RL input; V_CG input; accel_y_CG input; max_accel_y_cg input
function regen_en  = en_reg(V_RR, V_RL, V_CG, accel_y_CG, max_accel_y_cg)
    if(V_RR < 0.55 || V_RL < 0.55) % disable regen for speeds under 2kph to avoid
        regen_en = false;
        return;
    end
    if(V_CG >= 8 && accel_y_CG >= max_accel_y_cg) % disable regen while cornering to avoid disrupting balance
        regen_en = false;
        return;
    end
    regen_en = true;
    return;
end
